simulink model "sensorLib"  (R2020b)
settings: Solver=VariableStepAuto  StartTime=0.0  StopTime=10.0  RelTol=1e-3
undefined symbols (not defined in the file): States
libraries: sharedtransform x1, mspsensorlib x1
settings Model: Creator=dbell44  LastModifiedBy=dbell44

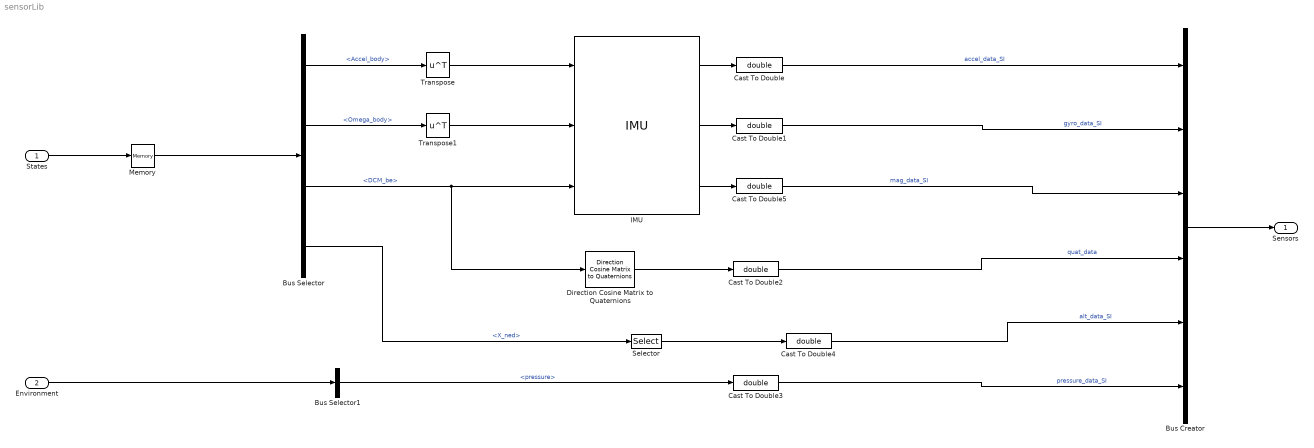
== system sensorLib ==
  States : Inport  OutDataTypeStr=Bus: StatesBus
  Environment : Inport  Port=2  OutDataTypeStr=Bus: EnvironmentBus
  Bus Creator : BusCreator  Inputs=6  OutDataTypeStr=Bus: SensorBus
  Bus Selector : BusSelector  OutputSignals=Accel_body,Omega_body,DCM_be,X_ned
  Bus Selector1 : BusSelector  OutputSignals=AtmosphereBus.pressure
  Cast To Double{,1..5} (6 alike) : DataTypeConversion  OutDataTypeStr=double
  Direction Cosine Matrix to Quaternions : sharedtransform/Direction Cosine Matrix  to Quaternions  aMode=0  action=None  tolerance=eps(2)
      settings: SourceProductBaseCode=AE,PW,MT,UV,VE,VP
  IMU : mspsensorlib/IMU  DispRefFrame=NED  Temperature=25  MagneticFieldNED=[ 27.5550, -2.4169, -16.0849 ]  MagneticFieldENU=[ -2.4169, 27.5550, 16.0849 ]  SeedDouble=67  SimulateUsing=Code generation  AccelParamsMeasurementRange=Inf  AccelParamsResolution=0  AccelParamsConstantBias=[ 0, 0, 0 ]  AccelParamsAxesMisalignment=[ 0, 0, 0 ]  AccelParamsNoiseDensity=[ 0, 0, 0 ]  AccelParamsBiasInstability=[ 0, 0, 0 ]  AccelParamsRandomWalk=[ 0, 0, 0 ]  AccelParamsTemperatureBias=[ 0, 0, 0 ]  AccelParamsTemperatureScaleFactor=[ 0, 0, 0 ]  GyroParamsMeasurementRange=Inf  GyroParamsResolution=0  GyroParamsConstantBias=[ 0, 0, 0 ]  GyroParamsAxesMisalignment=[ 0, 0, 0 ]  GyroParamsAccelerationBias=[ 0, 0, 0 ]  GyroParamsNoiseDensity=[ 0, 0, 0 ]  GyroParamsBiasInstability=[ 0, 0, 0 ]  GyroParamsRandomWalk=[ 0, 0, 0 ]  GyroParamsTemperatureBias=[ 0, 0, 0 ]  GyroParamsTemperatureScaleFactor=[ 0, 0, 0 ]  MagParamsMeasurementRange=Inf  MagParamsResolution=0  MagParamsConstantBias=[ 0, 0, 0 ]  MagParamsAxesMisalignment=[ 0, 0, 0 ]  MagParamsNoiseDensity=[ 0, 0, 0 ]  MagParamsBiasInstability=[ 0, 0, 0 ]  MagParamsRandomWalk=[ 0, 0, 0 ]  MagParamsTemperatureBias=[ 0, 0, 0 ]  MagParamsTemperatureScaleFactor=[ 0, 0, 0 ]
      settings: SourceProductBaseCode=TF,NV
  Memory : Memory  InitialCondition=States  InheritSampleTime=on
  Selector : Selector  InputPortWidth=3  IndexOptions=Index vector (dialog)  Indices=[3]  OutputSizes=1
  Transpose : Math  Operator=transpose  SaturateOnIntegerOverflow=on
  Transpose1 : Math  Operator=transpose  SaturateOnIntegerOverflow=on
  Sensors : Outport  OutDataTypeStr=Bus: SensorBus
  wires:
  Cast To Double3/1 -> Bus Creator/6  "pressure_data_SI"
  IMU/3 -> Cast To Double5/1
  States/1 -> Memory/1
  Transpose1/1 -> IMU/2
  Bus Selector/1 -> Transpose/1  "<Accel_body>"
  Cast To Double4/1 -> Bus Creator/5  "alt_data_SI"
  Bus Selector1/1 -> Cast To Double3/1  "<pressure>"
  Bus Creator/1 -> Sensors/1
  Memory/1 -> Bus Selector/1
  Environment/1 -> Bus Selector1/1
  Bus Selector/2 -> Transpose1/1  "<Omega_body>"
  Bus Selector/4 -> Selector/1  "<X_ned>"
  IMU/2 -> Cast To Double1/1
  Selector/1 -> Cast To Double4/1
  Direction Cosine Matrix to Quaternions/1 -> Cast To Double2/1
  IMU/1 -> Cast To Double/1
  Cast To Double5/1 -> Bus Creator/3  "mag_data_SI"
  Cast To Double2/1 -> Bus Creator/4  "quat_data"
  Transpose/1 -> IMU/1
  Cast To Double1/1 -> Bus Creator/2  "gyro_data_SI"
  Bus Selector/3 -> IMU/3, Direction Cosine Matrix to Quaternions/1  "<DCM_be>"
  Cast To Double/1 -> Bus Creator/1  "accel_data_SI"
